simulink model "intersection"  (R2021a)
settings: Solver=VariableStepAuto  StartTime=0.0  StopTime=10.0  RelTol=1e-3
values from neighbouring files (symbols this model uses):
  Ax = [X_RobotT(:);X_Robot1T(:);X_Robot2T(:)]    [path_obst.m]
  Ay = [Y_RobotT(:);Y_Robot1T(:);Y_Robot2T(:)]    [path_obst.m]
  Ox = obst(:,1)    [path_obst.m]
  Oy = obst(:,2)    [path_obst.m]

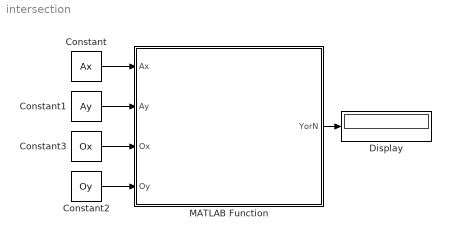
== system intersection ==
  Constant : Constant  Value=Ax
  Constant1 : Constant  Value=Ay
  Constant2 : Constant  Value=Oy
  Constant3 : Constant  Value=Ox
  Display : Display
  MATLAB Function : MATLAB Function  TreatAsAtomicUnit=on
  wires:
  Constant/1 -> MATLAB Function/1(Ax)
  Constant1/1 -> MATLAB Function/2(Ay)
  Constant2/1 -> MATLAB Function/4(Oy)
  Constant3/1 -> MATLAB Function/3(Ox)
  MATLAB Function/1(YorN) -> Display/1

== matlab function intersection/MATLAB Function ==
function YorN = fcn(Ax,Ay,Ox,Oy)
s1=size(Ax)/2;
s2=size(Ox)/2;
a1=zeros(s1(1),1);
b1=zeros(s1(1),1);
c1=zeros(s1(1),1);
a2=zeros(s2(1),1);
b2=zeros(s2(1),1);
c2=zeros(s2(1),1);
YorN=0;
for n=1:s1(1)
   a1(n) = Ay(2*n) - Ay(2*n-1);
   b1(n) = Ax(2*n-1) - Ax(2*n);
   c1(n) = a1(n)*Ax(2*n-1) + b1(n)*Ay(2*n-1);
end    
for i=1:s2(1)
   a2(i) = Oy(2*i) - Oy(2*i-1);
   b2(i) = Ox(2*i-1) - Ox(2*i);
   c2(i) = a2(i)*Ox(2*i-1) + b2(i)*Oy(2*i-1);
 end    
for i=1:s2(1)
    for n=1:s1(1)
        
     if (a1(n)*b2(i) - a2(i)*b1(n))==0
       X =inf;    
     else
       X =(b2(i)*c1(n) - b1(n)*c2(i))/(a1(n)*b2(i) - a2(i)*b1(n));
     end
     
     if X > max(Ax(2*n-1),Ax(2*n))|| X < min(Ax(2*n-1),Ax(2*n))|| X > max(Ox(2*i-1),Ox(2*i))|| X < min(Ox(2*i-1),Ox(2*i))
     else
          YorN=1;
     end
   end
end
